simulink model "Experiment_1_cs"  (Simulink 8.4)
settings: Solver=ode5  SolverMode=SingleTasking  StartTime=0.0  StopTime=inf  FixedStep=1/100  RelTol=1e-3
PreLoadFcn:
  | mbxruntime.callbacks.PreLoadFcn(bdroot);
PostLoadFcn:
  | mbxruntime.callbacks.PostLoadFcn(bdroot);
InitFcn:
  | mbxruntime.callbacks.InitFcn(bdroot);
StartFcn:
  | mbxruntime.callbacks.StartFcn(bdroot);
StopFcn:
  | mbxruntime.callbacks.StopFcn(bdroot);
undefined symbols (not defined in the file or in its folder): dfreq, gray, Rec, SDTV, strel
libraries: simulink x42, PreScanSimulinkLibrary x17, visiontextngfix x15, simulink_extras x12, visionconversions x3, PreScanUsefulBlocks x3, visionsinks x2, visionstatistics x1, visionmorphops x1, visionanalysis x1, simulink_need_slupdate x1
(part 8 of 8)

== matlab function Audi_A8_1/ENABLED/PPS Model/Pedestrian detection/Image processing/Embedded MATLAB Function ==
  data: im output double size=[375 500]; image input double
function im = sub_image(image)
%#eml
im=zeros(size(image,1),size(image,2));
for i=1:size(image,1)
    for j=1:size(image,2)
        if (image(i,j)==0)
            im(i,j)=1;
        else
            im(i,j)=0;
        end
    end
end

== matlab function Audi_A8_1/ENABLED/PPS Model/Pedestrian detection/PEDES ==
  data: CentAlarms output double; PosObj_subim input double; Centroid_subim input double; alarms output double size=TISdet; BBox input double; BBox_det output double; TISdet parameter double
function [CentAlarms,alarms,BBox_det]= pedes(PosObj_subim, Centroid_subim,BBox,TISdet)
%#eml
CentAlarms=int32(zeros(2,size(PosObj_subim,2)));
alarms=zeros(size(PosObj_subim,2),1);
BBox_det=int32(zeros(4,size(BBox,2)));
a=1;
for i=1:size(PosObj_subim,2)
    for j=1:size(Centroid_subim,2)
        if (Centroid_subim(1,j)~=0)||(Centroid_subim(2,j)~=0)
            if (abs(Centroid_subim(2,j)-PosObj_subim(2,i))<15)||(abs(Centroid_subim(1,j)-PosObj_subim(1,i))<15)%(PosObj_subim(1,i))>BBox(1,j)&&(PosObj_subim(1,i))<(BBox(1,j)+BBox(3,j))
                alarms(a,1)=1;
                CentAlarms(:,a)=PosObj_subim(:,i);%Centroid_subim(:,j);
                BBox_det(:,a)=BBox(:,i);
            end
        end
    end
    a=a+1;
end

== matlab function Audi_A8_1/ENABLED/PPS Model/Pedestrian detection/PEDES1 ==
  data: Im input double size=[375 500]; Imout output double size=[375 500 3]
function Imout = imag(Im)
%#eml
Imout=128*ones(size(Im,1),size(Im,2),3);
Imout(:,:,1)=Im;

== matlab function Audi_A8_1/ENABLED/PPS Model/Pedestrian detection/PEDES2 ==
  data: Im input double size=[375 500]; Imout output double size=[375 500 3]
function Imout = imag(Im)
%#eml
Imout=128*ones(size(Im,1),size(Im,2),3);
Imout(:,:,1)=Im;

== matlab function Audi_A8_1/ENABLED/PPS Model/Pedestrian detection/scaling_crop ==
  data: im input double; PosObj input double; X input double; Y input double; sub_im output double size=[375 500]; posObj_subim output double; im_x output double; im_y output double; liminf_x output double; liminf_y output double; rectangle output double
function [sub_im,posObj_subim,im_x,im_y,liminf_x, liminf_y,rectangle]=escaling(im,PosObj,X,Y)

minPx=size(im,2);
minPy=size(im,1);
maxPx=0;
maxPy=0;
detected=0;
mino=0;
maxo=0;
for i=1:size(PosObj,2)
    if PosObj(2,i)~=0
        if(PosObj(2,i)<minPx)
            minPx=PosObj(2,i);
            minPy=PosObj(1,i);
            mino=i;
        end
        if (PosObj(2,i)>maxPx)
            maxPx=PosObj(2,i);
            maxPy=PosObj(1,i);
            maxo=i;
        end
        detected=detected+1;
    end
end
if (detected==0)
    liminf_x=size(im,2);
    limsup_x=size(im,2);
    liminf_y=size(im,1);
    limsup_y=size(im,1);
 
 else
   
  %%For horizontal and vertical position
   
  if (mino~=0) 
    liminf_x= round(minPx-((40-round(1.6*Y(mino)))*2));
    liminf_y= round(minPy-((100-round(4.5*Y(mino)))*2));
    
  else
     liminf_x=1;
     liminf_y=1;
  end
   if (maxo~=0)   
    limsup_x= abs(round(maxPx+((40-round(1.6*Y(maxo)))*2)));
    limsup_y= abs(round(maxPy+((100-round(5*Y(maxo)))*2)));
   else
       limsup_x=size(im,2);
       limsup_y=size(im,1);
   end

end

  if (liminf_x<1)
         liminf_x=1;
  end
    
  if (limsup_x>size(im,2))
        limsup_x=size(im,2);
  end
    
  if (liminf_y<1)
       liminf_y=1;
  end
    
  if (limsup_y>=size(im,1))
       limsup_y=size(im,1);
  end
  
  if (liminf_y > size(im,1))
        liminf_y = size(im,1);
  end
    
   posObj_subim=zeros(2,size(PosObj,2));
   a=1;
    
    for i=1:size(PosObj,2)
        if (PosObj(2,i)~=0)
            posObj_subim(:,a)=[PosObj(1,i)-liminf_y;PosObj(2,i)-liminf_x];
            a=a+1;
        end
    end

sub_im=im(liminf_y:limsup_y,liminf_x:limsup_x);

if length( sub_im ) < 3
    sub_im = zeros(3,3,'uint8');
end


im_x=limsup_x-liminf_x;
im_y=limsup_y-liminf_y;
rectangle=[liminf_y liminf_x im_y im_x];

== matlab function Audi_A8_1/ENABLED/PPS Model/Radar detection/Straight road segment/Relative velocity2/Embedded MATLAB Function1 ==
  data: r input double; yp2 output double; yp1 input double; K1 input double; K2 output double; TISdet parameter double; TISMaxRange parameter double
function [yp2, K2] = modif(r, yp1, K1, TISdet, TISMaxRange)
%#eml
% Interpolating yp value.

K2 = K1;
yp2 = yp1;

d = 50;

% Adding point
for i = 1 : TISdet
   if r(i) ~= 150
      K2(i,1:d-1) = K2(i,2:d);
      K2(i,d) = yp1(i);
   end
end

% Choosing what to take
for i = 1 : TISdet
    s = 0;
    suma = 0;
    for j = 1 : 50
        if K2(i,j) ~= 0
            suma = suma + K2(i,j);
            s = s + 1;
        end
    end
    yp2(i) = suma/s;
end

% Returning, if object is not detected
for i = 1: TISdet
    if r(i) == TISMaxRange && yp1(i) == 0
        K2(i,:,:) = zeros(d,1);
        yp2(i) = 0;
    end    
end

== matlab function Audi_A8_1/ENABLED/PPS Model/Pedestrian detection/PEDES5 ==
  data: blob_subim_proces output double; sub_im input double size=[375 500]; limx_inf input double; limy_inf input double; im_x input double; im_y input double
function blob_subim_proces = blob_subim(sub_im, limx_inf, limy_inf,im_x,im_y)
%#eml
blob_subim_proces=single(zeros(375,500));

limx_sup=limx_inf+im_x;
limy_sup=limy_inf+im_y;

% Assigned the superior and inferior limit 
limx_sup_sorted=max([limx_sup limx_inf]);
limx_inf_sorted=min([limx_sup limx_inf]);
limy_inf_sorted=min([limy_sup limy_inf]);
limy_sup_sorted=max([limy_sup limy_inf]);


[nn, mm] = size( sub_im );
if ( nn <= 3 ) && ( mm <= 3 )
    sub_im = 0;
    % Create a zeros matrix of size (im_y,im_x)
    if im_x~=0 || im_y~=0
        im_x=abs(im_x);
        im_y=abs(im_y);
        assert(im_x<1000);
        assert(im_y<1000);
        sub_im=zeros(im_y+1,im_x+1);
    end
end


blob_subim_proces(limy_inf_sorted:limy_sup_sorted,limx_inf_sorted:limx_sup_sorted)=sub_im;

== matlab function Audi_A8_1/ENABLED/PPS Model/Radar detection/Straight road segment/Relative velocity2/Translation ==
  data: v input double; xpd input double; xp_dot output double; TISdet parameter double
function xp_dot = trans(v, xpd, TISdet)
%#codegen
%Translation of the value

xp_dot = xpd;
for i = 1 : TISdet
    if xpd(i) == v
        xp_dot(i) =0;
    end
end
end

== matlab function Audi_A8_1/ENABLED/PPS Model/Radar detection/Straight road segment/THETA Derivative1/Deriv correction ==
  data: th input double; thp input double; thd input double; th_dot output double; TISdet parameter double
function th_dot = stopping(th, thp, thd, TISdet)
%#codegen
% Stopping if nothing is detected.

th_dot = thd;
for i = 1 : TISdet
    if (th(i)==0 && thp(i)~=0) || (th(i)~=0 && thp(i)==0)
        th_dot(i) = 0;
    end
end
end

== matlab function BMW_Z3_1/ENABLED/MATLAB Function ==
  data: carX input double; pedResultX output double; carY input double; carZ input double; carRotZ input double; pedR input double; pedTheta input double; pedPhi input double; sensorCorrX input double; sensorCorrY input double; sensorCorrZ input double; pedResultY output double; pedResultZ output double
function [pedResultX,pedResultY,pedResultZ] = calculatePositionFunc(carX,carY,carZ,carRotZ,pedR,pedTheta,pedPhi,sensorCorrX,sensorCorrY,sensorCorrZ)

[xPed,yPed,zPed] = sph2cart(-pedTheta*pi/180,pedPhi*pi/180,pedR);

TcarMat = [1 0 0 carX ; 0 1 0 carY ; 0 0 1 carZ ; 0 0 0 1];

TpedMat = [1 0 0 xPed ; 0 1 0 yPed ; 0 0 1 zPed ; 0 0 0 1];

TsensorMat = [1 0 0 sensorCorrX ; 0 1 0 sensorCorrY ; 0 0 1 sensorCorrZ ; 0 0 0 1];

RcarMat = [cosd(carRotZ) -sind(carRotZ) 0 0 ;
    sind(carRotZ) cosd(carRotZ) 0 0;
    0 0 1 0;
    0 0 0 1];



ResultMat = TcarMat*RcarMat*TsensorMat*TpedMat*[0;0;0;1];

pedResultX = ResultMat(1);
pedResultY = ResultMat(2);
pedResultZ = ResultMat(3);

== matlab function Audi_A8_1/ENABLED/MATLAB Function2 ==
  data: carX input double; pedR output double; carY input double; carZ input double; carRotZ input double; pedX input double; pedY input double; pedZ input double; sensorCorrX input double; sensorCorrY input double; sensorCorrZ input double; pedTheta output double; pedPhi output double
function [pedR,pedTheta,pedPhi] = calculateTISdataFunc(carX,carY,carZ,carRotZ,pedX,pedY,pedZ,sensorCorrX,sensorCorrY,sensorCorrZ)
%#codegen
TcarMat = [1 0 0 carX ; 0 1 0 carY ; 0 0 1 carZ ; 0 0 0 1];

RcarMat = [cosd(carRotZ) -sind(carRotZ) 0 0;
    sind(carRotZ) cosd(carRotZ) 0 0;
    0 0 1 0;
    0 0 0 1];

TsensorMat = [1 0 0 sensorCorrX ; 0 0 1 sensorCorrY ; 0 1 0 sensorCorrZ ; 0 0 0 1];

FcarMat = TcarMat*RcarMat*TsensorMat*[0;0;0;1];

[pedThetaTemp,pedPhiTemp,pedRTemp] = cart2sph(pedX - FcarMat(1), pedY - FcarMat(2), pedZ - FcarMat(3));

pedR = pedRTemp;
pedTheta = -(pedThetaTemp*180/pi-carRotZ);
pedPhi = pedPhiTemp*180/pi;

== matlab function Audi_A8_1/ENABLED/MATLAB Function ==
  data: pedR input double; pedR_Array output double; pedTheta input double; dVel input double; pedTheta_Array output double; dVel_Array output double
function [pedR_Array,pedTheta_Array,dVel_Array] = fcn(pedR,pedTheta,dVel)

pedR_Array = zeros(32,1);
pedTheta_Array = zeros(32,1);
dVel_Array = zeros(32,1);

pedR_Array(1) = pedR(1);
pedTheta_Array(1) = pedTheta(1);
dVel_Array(1) = dVel(1);

pedR_Array(2) = pedR(2);
pedTheta_Array(2) = pedTheta(2);
dVel_Array(2) = dVel(2);

== matlab function BMW_Z3_1/ENABLED/MATLAB Function3 ==
  data: carAngle input double; carVelocity input double; dTranslationX output double; dopplerTX input double; dopplerTY input double; dTranslationY output double
function [dTranslationX,dTranslationY] = globalAxisConversion(carAngle,carVelocity,dopplerTX,dopplerTY)

rotMat = [cosd(carAngle) -sind(carAngle);
    sind(carAngle) cosd(carAngle)];

carVelX = carVelocity*cosd(carAngle);
carVelY = carVelocity*sind(carAngle);

carVelMat = [carVelX ; carVelY];

Vdv = rotMat*[dopplerTX;dopplerTY];

Vdv = Vdv + carVelMat;

dTranslationX = Vdv(1);
dTranslationY = Vdv(2);

== matlab function Audi_A8_1/ENABLED/MATLAB Function1 ==
  data: carX input double; dopplerVelocity output double; carY input double; carZ input double; carAngle input double; carVelocity input double; pedX input double; pedY input double; pedZ input double; dTranslationX input double; dTranslationY input double; dTranslationZ input double; sensorX input double; sensorY input double; sensorZ input double
function dopplerVelocity = relativeVelocity(carX,carY,carZ,carAngle,carVelocity,pedX,pedY,pedZ,dTranslationX,dTranslationY,dTranslationZ,sensorX,sensorY,sensorZ)

rotMat = [cosd(carAngle) -sind(carAngle);
    sind(carAngle) cosd(carAngle)];

sensorMat = rotMat*[sensorX ; sensorY];

carVelX = carVelocity*cosd(carAngle);
carVelY = carVelocity*sind(carAngle);

carVelMat = rotMat\[carVelX ; carVelY];

carMat = [carX + sensorMat(1) ; carY + sensorMat(2)];

Vcp = [pedX - carMat(1) ; pedY - carMat(2)];

Vdv = rotMat\[dTranslationX ; dTranslationY];

Vdv = Vdv - carVelMat;

Vcp = rotMat\Vcp;

dopplerVelocity = dot(Vdv,Vcp)/norm(Vcp);
